simulink model "untitled"  (R2022a)
settings: Solver=VariableStepAuto  StartTime=0.0  StopTime=100  RelTol=1e-3
libraries: simulink x6
settings Model: Creator=Adarsh  LastModifiedBy=Adarsh

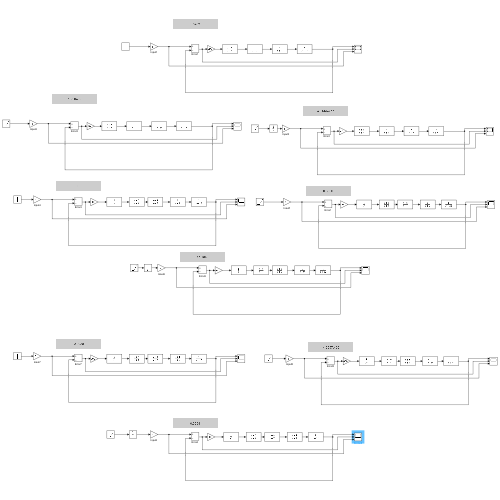
[thumbnail: Simulink's stored preview of the top-level diagram]
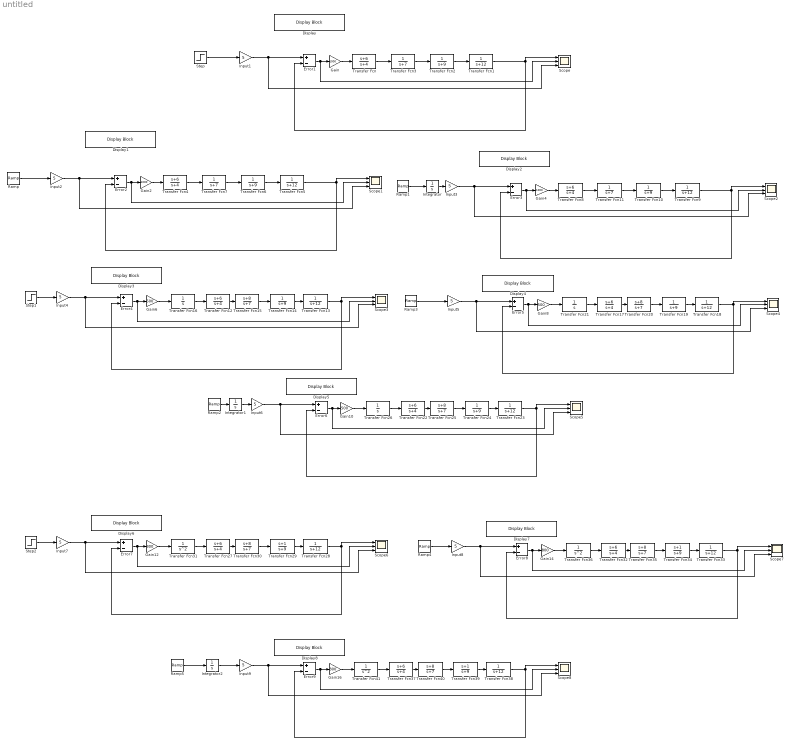
== system untitled ==
  Display{,1..8} (9 alike) : DisplayBlock  LabelPosition=Hide  Transparency=1
  Error{1..9} (9 alike) : Sum  Inputs=+-
  Gain : Gain  Gain=1000
  Gain10 : Gain  Gain=500
  Gain12 : Gain  Gain=800
  Gain14 : Gain  Gain=800
  Gain16 : Gain  Gain=800
  Gain2 : Gain  Gain=1000
  Gain4 : Gain  Gain=1000
  Gain6 : Gain  Gain=500
  Gain8 : Gain  Gain=500
  Input{1..9} (9 alike) : Gain  Gain=5
  Integrator : Integrator
  Integrator1 : Integrator
  Integrator2 : Integrator
  Ramp{,1..5} (6 alike) : simulink/Sources/Ramp  slope=1  start=0  InitialOutput=0
  Scope{,1..8} (9 alike) : Scope  NumInputPorts=3
  Step : Step  SampleTime=0
  Step1 : Step  SampleTime=0
  Step2 : Step  SampleTime=0
  Transfer Fcn{,4,8,12,17,22,27,32,37} (9 alike) : TransferFcn  Numerator=[1 6]  Denominator=[1 4]
  Transfer Fcn{1,5,9,13,18,23,28,33,38} (9 alike) : TransferFcn  Denominator=[1 12]
  Transfer Fcn{2,6,10,14,19,24} (6 alike) : TransferFcn  Denominator=[1 9]
  Transfer Fcn11 : TransferFcn  Denominator=[1 7]
  Transfer Fcn{15,20,25,30,35,40} (6 alike) : TransferFcn  Numerator=[1 8]  Denominator=[1 7]
  Transfer Fcn16 : TransferFcn  Denominator=[1 0]
  Transfer Fcn21 : TransferFcn  Denominator=[1 0]
  Transfer Fcn26 : TransferFcn  Denominator=[1 0]
  Transfer Fcn29 : TransferFcn  Numerator=[1 1]  Denominator=[1 9]
  Transfer Fcn3 : TransferFcn  Denominator=[1 7]
  Transfer Fcn31 : TransferFcn  Denominator=[1 0 0]
  Transfer Fcn34 : TransferFcn  Numerator=[1 1]  Denominator=[1 9]
  Transfer Fcn36 : TransferFcn  Denominator=[1 0 0]
  Transfer Fcn39 : TransferFcn  Numerator=[1 1]  Denominator=[1 9]
  Transfer Fcn41 : TransferFcn  Denominator=[1 0 0]
  Transfer Fcn7 : TransferFcn  Denominator=[1 7]
  wires:
  Gain/1 -> Transfer Fcn/1
  Transfer Fcn/1 -> Transfer Fcn3/1
  Transfer Fcn3/1 -> Transfer Fcn2/1
  Transfer Fcn2/1 -> Transfer Fcn1/1
  Transfer Fcn1/1 -> Scope/1, Error1/2
  Step/1 -> Input1/1
  Error1/1 -> Scope/2, Gain/1
  Input1/1 -> Scope/3, Error1/1
  Transfer Fcn6/1 -> Transfer Fcn5/1
  Gain2/1 -> Transfer Fcn4/1
  Transfer Fcn4/1 -> Transfer Fcn7/1
  Transfer Fcn5/1 -> Scope1/1, Error2/2
  Input2/1 -> Scope1/3, Error2/1
  Transfer Fcn7/1 -> Transfer Fcn6/1
  Error2/1 -> Scope1/2, Gain2/1
  Ramp/1 -> Input2/1
  Transfer Fcn10/1 -> Transfer Fcn9/1
  Gain4/1 -> Transfer Fcn8/1
  Transfer Fcn8/1 -> Transfer Fcn11/1
  Transfer Fcn9/1 -> Scope2/1, Error3/2
  Input3/1 -> Scope2/3, Error3/1
  Transfer Fcn11/1 -> Transfer Fcn10/1
  Error3/1 -> Scope2/2, Gain4/1
  Integrator/1 -> Input3/1
  Ramp1/1 -> Integrator/1
  Input4/1 -> Scope3/3, Error4/1
  Transfer Fcn13/1 -> Scope3/1, Error4/2
  Transfer Fcn14/1 -> Transfer Fcn13/1
  Error4/1 -> Scope3/2, Gain6/1
  Transfer Fcn15/1 -> Transfer Fcn14/1
  Transfer Fcn12/1 -> Transfer Fcn15/1
  Transfer Fcn16/1 -> Transfer Fcn12/1
  Gain6/1 -> Transfer Fcn16/1
  Transfer Fcn17/1 -> Transfer Fcn20/1
  Gain8/1 -> Transfer Fcn21/1
  Transfer Fcn20/1 -> Transfer Fcn19/1
  Error5/1 -> Scope4/2, Gain8/1
  Input5/1 -> Scope4/3, Error5/1
  Transfer Fcn18/1 -> Scope4/1, Error5/2
  Ramp3/1 -> Input5/1
  Transfer Fcn21/1 -> Transfer Fcn17/1
  Transfer Fcn19/1 -> Transfer Fcn18/1
  Step1/1 -> Input4/1
  Transfer Fcn22/1 -> Transfer Fcn25/1
  Gain10/1 -> Transfer Fcn26/1
  Transfer Fcn25/1 -> Transfer Fcn24/1
  Error6/1 -> Scope5/2, Gain10/1
  Input6/1 -> Scope5/3, Error6/1
  Transfer Fcn23/1 -> Scope5/1, Error6/2
  Transfer Fcn26/1 -> Transfer Fcn22/1
  Transfer Fcn24/1 -> Transfer Fcn23/1
  Ramp2/1 -> Integrator1/1
  Integrator1/1 -> Input6/1
  Transfer Fcn27/1 -> Transfer Fcn30/1
  Gain12/1 -> Transfer Fcn31/1
  Transfer Fcn30/1 -> Transfer Fcn29/1
  Error7/1 -> Scope6/2, Gain12/1
  Input7/1 -> Scope6/3, Error7/1
  Transfer Fcn28/1 -> Scope6/1, Error7/2
  Transfer Fcn31/1 -> Transfer Fcn27/1
  Step2/1 -> Input7/1
  Transfer Fcn29/1 -> Transfer Fcn28/1
  Transfer Fcn32/1 -> Transfer Fcn35/1
  Gain14/1 -> Transfer Fcn36/1
  Transfer Fcn35/1 -> Transfer Fcn34/1
  Error8/1 -> Scope7/2, Gain14/1
  Input8/1 -> Scope7/3, Error8/1
  Transfer Fcn33/1 -> Scope7/1, Error8/2
  Transfer Fcn36/1 -> Transfer Fcn32/1
  Transfer Fcn34/1 -> Transfer Fcn33/1
  Transfer Fcn37/1 -> Transfer Fcn40/1
  Gain16/1 -> Transfer Fcn41/1
  Transfer Fcn40/1 -> Transfer Fcn39/1
  Error9/1 -> Scope8/2, Gain16/1
  Input9/1 -> Scope8/3, Error9/1
  Transfer Fcn38/1 -> Scope8/1, Error9/2
  Transfer Fcn41/1 -> Transfer Fcn37/1
  Transfer Fcn39/1 -> Transfer Fcn38/1
  Ramp4/1 -> Input8/1
  Ramp5/1 -> Integrator2/1
  Integrator2/1 -> Input9/1
